simulink model "sampleModel2076_3_sub_sub"  (R2023a)
settings: Solver=VariableStepAuto  StartTime=0.0  StopTime=10.0  RelTol=1e-3
libraries: hdlsllib x6, simulink x1
settings Model: Creator=user1  LastModifiedBy=user1
settings OptimizationCC: BlockReduction=off  ConditionallyExecuteInputs=off

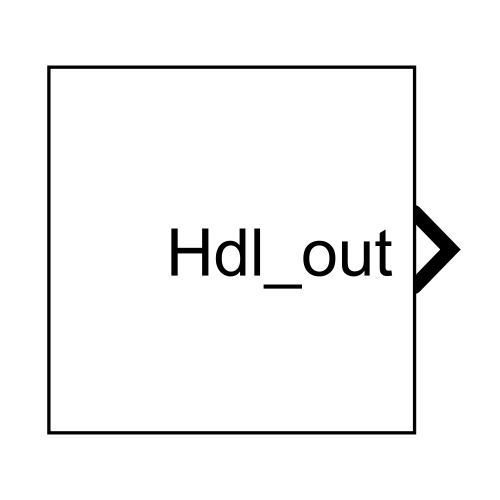
[thumbnail: Simulink's stored preview of the top-level diagram]
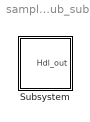
== system sampleModel2076_3_sub_sub ==
  Subsystem : Subsystem

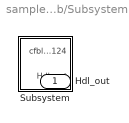
== system sampleModel2076_3_sub_sub/Subsystem ==
  Subsystem : Subsystem
  Hdl_out : Outport  OutDataTypeStr=uint8

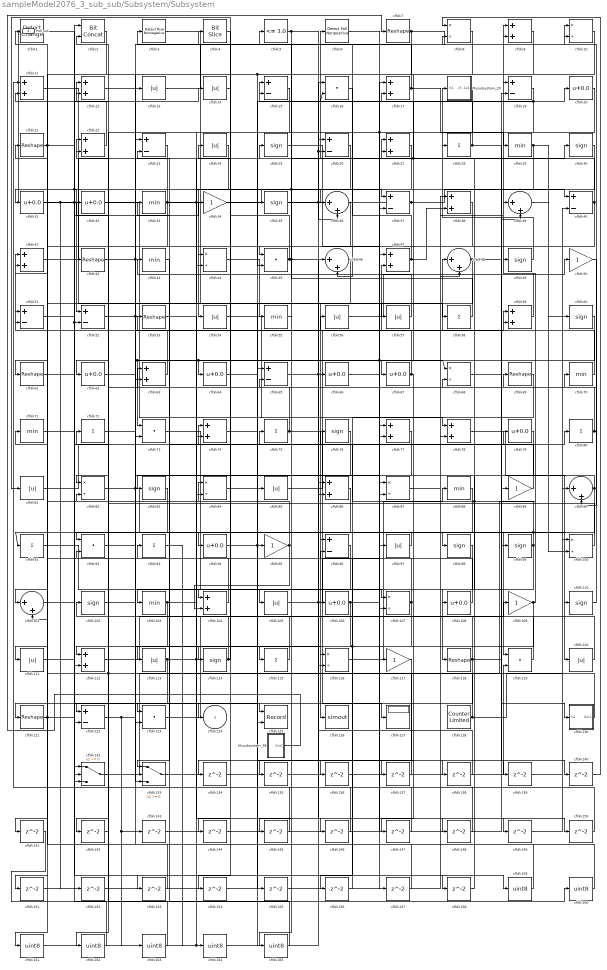
== system sampleModel2076_3_sub_sub/Subsystem/Subsystem ==
  Mysubsystem_20 : Subsystem  TreatAsAtomicUnit=on  RTWFcnName=Mysubsystem_20
      settings: RTWFcnNameOpts=User specified  RTWFileNameOpts=Use function name
  Mysubsystem_38 : Subsystem  TreatAsAtomicUnit=on  RTWFcnName=Mysubsystem_38
      settings: RTWFcnNameOpts=User specified  RTWFileNameOpts=Use function name
  cfblk1 : simulink/Logic and Bit Operations/Detect Change  vinit=0  OutDataTypeStr=uint8
      settings: LibrarySourceBlock=|
      | hdlsllib/Logic and Bit
      | Operations/Detect
      | Change
  cfblk{8,10,44,68,82,84,87,100,107,116} (10 alike) : Product  Inputs=*/  OutDataTypeStr=uint8  RndMeth=Zero  SaturateOnIntegerOverflow=on
  cfblk{36,39,46,48,90,101} (6 alike) : Sum  Inputs=|++  OutDataTypeStr=uint8
  cfblk{25,30,35,49,60,76,83,98..99,102,110,114} (12 alike) : Signum
  cfblk{29,33,43,55,70..71,88,103} (8 alike) : MinMax  OutDataTypeStr=uint8
  cfblk{9,11..12,17,22,27,38,41,47,59,63,74,77..78,86,104,112} (17 alike) : Sum  OutDataTypeStr=uint8
  cfblk{13..14,24,54,56..57,81,85,97,105,111,113,120} (13 alike) : Abs  OutDataTypeStr=uint8  SaturateOnIntegerOverflow=off
  cfblk{20,31..32,62,64,66..67,79,94,106,108} (11 alike) : Bias  Bias=0.0  SaturateOnIntegerOverflow=off
  cfblk{34,50,89,95,109,117} (6 alike) : Gain  OutDataTypeStr=uint8
  cfblk{28,58,72,75,80,91,93,115} (8 alike) : Sum  Inputs=+  OutDataTypeStr=uint8
  cfblk{7,21,42,53,61,69,118,121} (8 alike) : Reshape
  cfblk{16,45,73,92,119,123} (6 alike) : DotProduct  OutDataTypeStr=uint8
  cfblk{15,19,23,26,37,40,51..52,65,96,122} (11 alike) : Sum  Inputs=+-  OutDataTypeStr=uint8
  cfblk125 : Record  FileSettingsInternal="{\"entries\":[{\"content\":{\"excelSettings\":{\"content\":{},\"type\":\"Streamout.ExcelSettings\"}},\"type\":\"Streamout.FileSettingStorage\",\"uuid\":\"\"}],\"packageUris\":[\"http:\\/\\/schema.mathworks.com\\/mf0\\/streamout_blocks\\/R2020a\"],\"version\":\"1.0\"}"  Layout=[1 1]  SignalsInternal="{\"entries\":[{\"content\":{\"signals\":[{\"content\":{\"blockPath\":[],\"dimensions\":[1],\"domain\":\"\",\"lineColor\":\"#a2142f\",\"plots\":[1],\"port\":1,\"signalID\":61490,\"signalName\":\"cfblk5\"},\"type\":\"RecordBlkView.Signal\",\"uuid\":\"\"},{\"content\":{\"blockPath\":[],\"dimensions\":[1],\"domain\":\"\",\"lineColor\":\"#139fff\",\"plots\":[1],\"port\":2,\"signalID\":61493,\"signalName\":\"cfblk21\"},\"type\":\"RecordBlkView.Signal\",\"uuid\":\"\"}]},\"type\":\"RecordBlkView.InputSignals\",\"uuid\":\"\"}],\"packageUris\":[\"http:\\/\\/schema.mathworks.com\\/mf0\\/streamout_blocks\\/R2020a\"],\"version\":\"1.0\"}"  VisualizationBindings="{\"xyplotplugin\":{\"info\":[{\"series\":[{\"bindingParametersList\":[{\"parameter\":\"X-Axis\",\"signalID\":61490,\"signalName\":\"cfblk5\"},{\"parameter\":\"Y-Axis\",\"signalID\":61493,\"signalName\":\"cfblk21\"}],\"seriesID\":40952}],\"subplotID\":1}]}}"  CompatibilityTag=XY  st=-1
  cfblk126 : ToWorkspace  VariableName=simout  SaveFormat=Timeseries  SampleTime=-1
  cfblk127 : Display
  cfblk128 : hdlsllib/Sources/Counter Limited  uplimit=7  tsamp=-1
  cfblk130 : Subsystem
      settings: LibrarySourceBlock=|
      | hdlsllib/Ports &
      | Subsystems/Subsystem
  cfblk132 : Switch  OutDataTypeStr=uint8  SaturateOnIntegerOverflow=off  InputSameDT=off
  cfblk133 : Switch  OutDataTypeStr=uint8  SaturateOnIntegerOverflow=off  InputSameDT=off
  cfblk{134..158} (25 alike) : Delay  SampleTime=1
  cfblk{159..165} (7 alike) : DataTypeConversion  OutDataTypeStr=uint8  SaturateOnIntegerOverflow=off  RndMeth=Floor
  cfblk2 : hdlsllib/Logic and Bit Operations/Bit Concat  numInputs=2
  cfblk3 : hdlsllib/Logic and Bit Operations/Detect Rise Nonnegative  vinit=0  OutDataTypeStr=uint8
  cfblk4 : hdlsllib/Logic and Bit Operations/Bit Slice  lidx=7  ridx=0
  cfblk5 : hdlsllib/Logic and Bit Operations/Compare To Constant  relop=<=  const=3.0  OutDataTypeStr=uint8
  cfblk6 : hdlsllib/Logic and Bit Operations/Detect Fall Nonpositive  vinit=0  OutDataTypeStr=uint8
  cfblk124 : Outport  OutDataTypeStr=uint8  VectorParamsAs1DForOutWhenUnconnected=off
  Hdl_out : Outport  Port=2  OutDataTypeStr=uint8
  wires:
  Mysubsystem_38/1(Out1) -> cfblk7/1
  Mysubsystem_20/1(cfblk124) -> cfblk124/1
  cfblk49/1 -> Mysubsystem_20/1(In1)
  cfblk165/1 -> cfblk93/1
  cfblk76/1 -> cfblk165/1
  cfblk164/1 -> cfblk26/2, cfblk16/1, cfblk106/1
  cfblk163/1 -> cfblk2/2
  cfblk162/1 -> cfblk2/1
  cfblk161/1 -> cfblk84/2, cfblk95/1
  cfblk160/1 -> cfblk1/1
  cfblk141/1 -> cfblk160/1
  cfblk159/1 -> cfblk32/1
  cfblk1/1 -> cfblk159/1
  cfblk158/1 -> cfblk28/1
  cfblk51/1 -> cfblk158/1
  cfblk157/1 -> cfblk21/1
  cfblk66/1 -> cfblk157/1
  cfblk156/1 -> cfblk96/2
  cfblk155/1 -> cfblk46/1
  cfblk64/1 -> cfblk155/1
  cfblk154/1 -> cfblk38/1
  cfblk14/1 -> cfblk154/1
  cfblk153/1 -> cfblk133/2
  cfblk152/1 -> cfblk48/2
  cfblk151/1 -> cfblk74/2
  cfblk150/1 -> cfblk92/2
  cfblk149/1 -> cfblk40/2
  cfblk148/1 -> cfblk65/1
  cfblk147/1 -> cfblk101/2
  cfblk146/1 -> cfblk23/1
  cfblk53/1 -> cfblk146/1
  cfblk145/1 -> cfblk11/1
  cfblk144/1 -> cfblk39/2
  cfblk143/1 -> cfblk37/2
  cfblk142/1 -> cfblk22/2
  cfblk15/1 -> cfblk142/1
  cfblk140/1 -> cfblk8/1
  cfblk68/1 -> cfblk140/1
  cfblk139/1 -> cfblk90/1
  cfblk138/1 -> cfblk86/1
  cfblk84/1 -> cfblk138/1
  cfblk137/1 -> cfblk47/1
  cfblk88/1 -> cfblk137/1
  cfblk136/1 -> cfblk78/2
  cfblk69/1 -> cfblk136/1
  cfblk135/1 -> cfblk119/2
  cfblk55/1 -> cfblk135/1
  cfblk134/1 -> cfblk19/2
  cfblk117/1 -> cfblk134/1
  cfblk44/1 -> cfblk55/1
  cfblk27/1 -> cfblk45/1, cfblk144/1
  cfblk112/1 -> cfblk109/1
  cfblk96/1 -> cfblk133/1
  cfblk113/1 -> cfblk27/1, cfblk150/1, cfblk151/1
  cfblk54/1 -> cfblk86/2
  cfblk65/1 -> cfblk26/1, cfblk149/1
  cfblk50/1 -> cfblk90/2
  cfblk94/1 -> cfblk116/2, cfblk59/2
  cfblk33/1 -> cfblk58/1, cfblk36/1, cfblk101/1, cfblk31/1
  cfblk2/1 -> cfblk161/1
  cfblk8/1 -> cfblk52/2, cfblk112/2, cfblk45/2
  cfblk119/1 -> cfblk74/1
  cfblk108/1 -> cfblk51/2
  cfblk99/1 -> cfblk76/1, cfblk68/2, cfblk91/1, cfblk108/1
  cfblk89/1 -> cfblk23/2
  cfblk13/1 -> cfblk8/2
  cfblk118/1 -> cfblk24/1, cfblk132/3, cfblk80/1
  cfblk61/1 -> cfblk132/1
  cfblk128/1 -> cfblk51/1, cfblk82/2, cfblk100/1
  cfblk93/1 -> cfblk164/1
  cfblk36/1 -> cfblk63/2
  cfblk29/1 -> cfblk61/1, cfblk132/2, cfblk100/2
  cfblk58/1 -> cfblk15/1
  cfblk12/1 -> cfblk114/1
  cfblk106/1 -> cfblk112/1, cfblk59/1
  cfblk63/1 -> cfblk41/1
  cfblk28/1 -> cfblk99/1, cfblk5/1
  cfblk130/1(Out1) -> cfblk33/1
  cfblk121/1 -> cfblk79/1, cfblk141/1
  cfblk16/1 -> cfblk46/2
  cfblk98/1 -> cfblk118/1
  cfblk31/1 -> cfblk14/1, cfblk153/1, cfblk152/1
  cfblk6/1 -> cfblk68/1, cfblk139/1
  cfblk87/1 -> cfblk39/1
  cfblk74/1 -> cfblk19/1
  cfblk46/1 -> cfblk82/1
  cfblk20/1 -> cfblk44/2
  cfblk104/1 -> cfblk71/1
  cfblk42/1 -> cfblk66/1, cfblk30/1
  cfblk122/1 -> cfblk143/1, cfblk163/1, cfblk27/2
  cfblk23/1 -> cfblk62/1
  cfblk37/1 -> cfblk40/1, Hdl_out/1
  cfblk26/1 -> cfblk122/2
  cfblk47/1 -> cfblk3/1, cfblk38/2
  cfblk67/1 -> cfblk53/1, cfblk147/1
  cfblk4/1 -> cfblk94/1
  cfblk10/1 -> cfblk115/1
  cfblk111/1 -> cfblk42/1
  cfblk83/1 -> cfblk122/1
  cfblk105/1 -> cfblk17/1
  cfblk100/1 -> cfblk12/1
  cfblk71/1 -> cfblk98/1
  cfblk19/1 -> cfblk105/1, cfblk77/2, cfblk16/2
  cfblk78/1 -> cfblk110/1
  cfblk41/1 -> cfblk6/1
  cfblk5/1 -> cfblk125/1, cfblk36/2
  cfblk109/1 -> cfblk156/1, cfblk162/1, cfblk49/1
  cfblk7/1 -> cfblk9/2, cfblk133/3
  cfblk80/1 -> cfblk10/1, cfblk12/2
  cfblk40/1 -> cfblk17/2, cfblk15/2, cfblk57/1
  cfblk43/1 -> cfblk123/1
  cfblk73/1 -> cfblk107/2
  cfblk57/1 -> cfblk43/1
  cfblk22/1 -> cfblk11/2
  cfblk48/1 -> cfblk121/1, cfblk130/1(In1)
  cfblk35/1 -> cfblk117/1, cfblk20/1
  cfblk97/1 -> cfblk96/1
  cfblk101/1 -> cfblk34/1
  cfblk107/1 -> cfblk22/1, cfblk123/2
  cfblk85/1 -> cfblk48/1
  cfblk114/1 -> cfblk102/1, cfblk84/1
  cfblk81/1 -> cfblk35/1
  cfblk24/1 -> cfblk44/1
  cfblk56/1 -> cfblk50/1
  cfblk11/1 -> cfblk85/1
  cfblk120/1 -> cfblk72/1
  cfblk21/1 -> cfblk111/1, cfblk125/2
  cfblk59/1 -> cfblk9/1
  cfblk62/1 -> cfblk13/1
  cfblk102/1 -> cfblk116/1
  cfblk32/1 -> cfblk97/1
  cfblk72/1 -> cfblk25/1
  cfblk133/1 -> cfblk89/1
  cfblk75/1 -> cfblk127/1, cfblk65/2
  cfblk25/1 -> cfblk87/1
  cfblk103/1 -> cfblk75/1, cfblk113/1
  cfblk115/1 -> cfblk63/1
  cfblk52/1 -> cfblk78/1, cfblk87/2
  cfblk60/1 -> cfblk73/1, cfblk73/2, cfblk64/1
  cfblk92/1 -> cfblk56/1
  cfblk70/1 -> cfblk47/2
  cfblk82/1 -> cfblk120/1, cfblk10/2
  cfblk123/1 -> cfblk77/1
  cfblk91/1 -> cfblk107/1
  cfblk86/1 -> cfblk92/1
  cfblk17/1 -> cfblk81/1, cfblk29/1
  cfblk39/1 -> cfblk60/1
  cfblk3/1 -> cfblk126/1
  cfblk132/1 -> cfblk69/1
  cfblk95/1 -> cfblk104/2, cfblk41/2
  cfblk116/1 -> cfblk88/1
  cfblk30/1 -> cfblk52/1
  cfblk77/1 -> cfblk103/1
  cfblk79/1 -> cfblk104/1
  cfblk110/1 -> cfblk70/1
  cfblk90/1 -> cfblk119/1, cfblk83/1
  cfblk45/1 -> cfblk145/1, cfblk148/1, cfblk4/1
  cfblk38/1 -> cfblk54/1
  cfblk9/1 -> cfblk67/1
  cfblk34/1 -> cfblk37/1

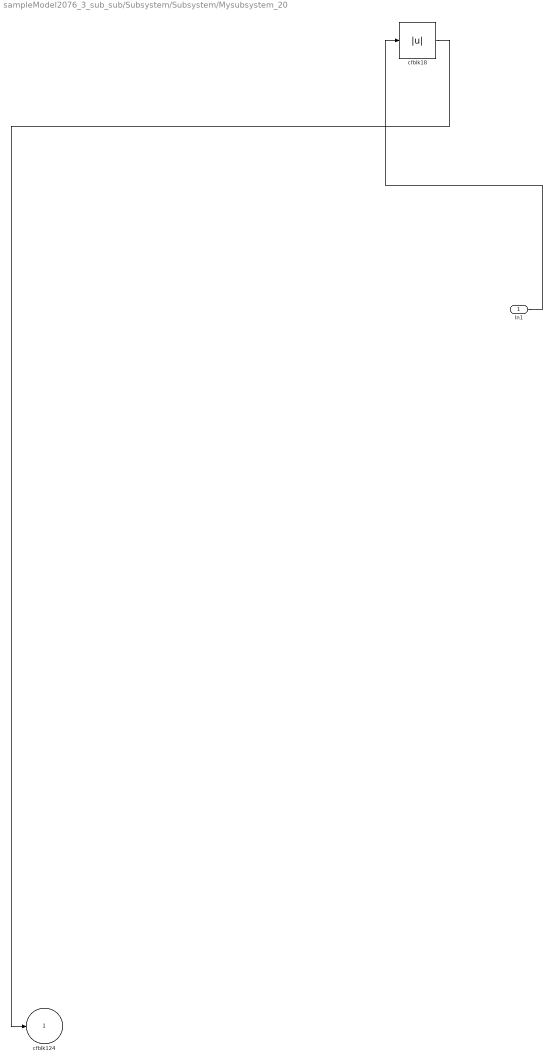
== system sampleModel2076_3_sub_sub/Subsystem/Subsystem/Mysubsystem_20 ==
  In1 : Inport
  cfblk18 : Abs  SaturateOnIntegerOverflow=off
  cfblk124 : Outport  VectorParamsAs1DForOutWhenUnconnected=off
  wires:
  cfblk18/1 -> cfblk124/1
  In1/1 -> cfblk18/1

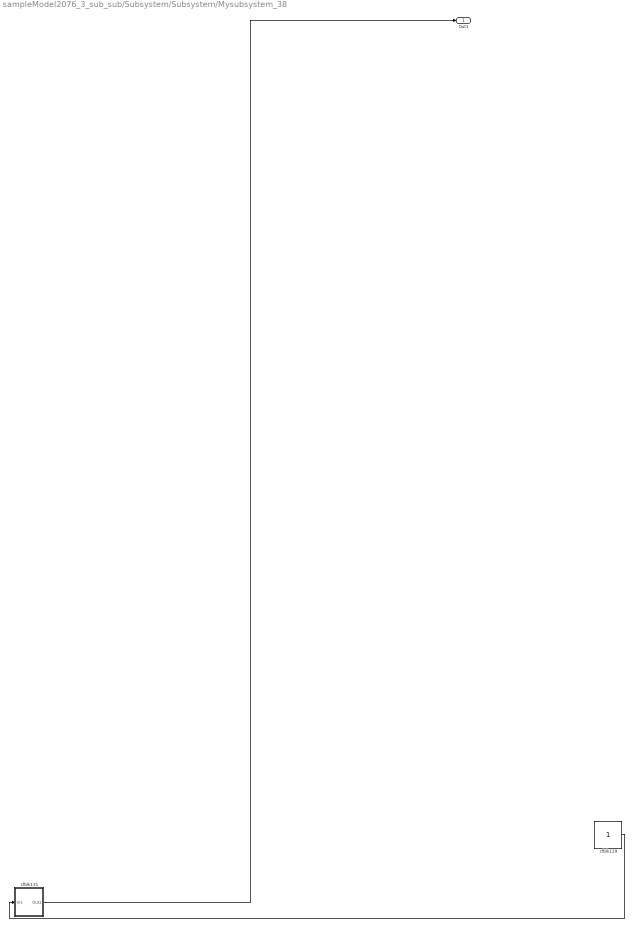
== system sampleModel2076_3_sub_sub/Subsystem/Subsystem/Mysubsystem_38 ==
  cfblk129 : Constant  SampleTime=-1
  cfblk131 : Subsystem
      settings: LibrarySourceBlock=|
      | hdlsllib/Ports &
      | Subsystems/Subsystem
  Out1 : Outport
  wires:
  cfblk131/1(Out1) -> Out1/1
  cfblk129/1 -> cfblk131/1(In1)

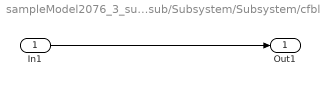
== system sampleModel2076_3_sub_sub/Subsystem/Subsystem/cfblk130 ==
  In1 : Inport
  Out1 : Outport
  wires:
  In1/1 -> Out1/1

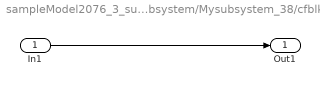
== system sampleModel2076_3_sub_sub/Subsystem/Subsystem/Mysubsystem_38/cfblk131 ==
  In1 : Inport
  Out1 : Outport
  wires:
  In1/1 -> Out1/1
